simulink model "binary_counter"  (R2022b)
settings: Solver=VariableStepAuto  StartTime=0.0  StopTime=inf  RelTol=1e-3
libraries: simulink_extras x5
settings Model: PacingRate=0.900000  Creator=F1  LastModifiedBy=Namratha
settings SolverCC: AlgebraicLoopSolver=TrustRegion
settings OptimizationCC: BooleanDataType=off
settings DebuggingCC: UnconnectedInputMsg=warning  UnconnectedOutputMsg=warning  UnconnectedLineMsg=warning  SFMachineParentedDataDiag=warning
settings ModelReferenceCC: EnableRefExpFcnMdlSchedulingChecks=on

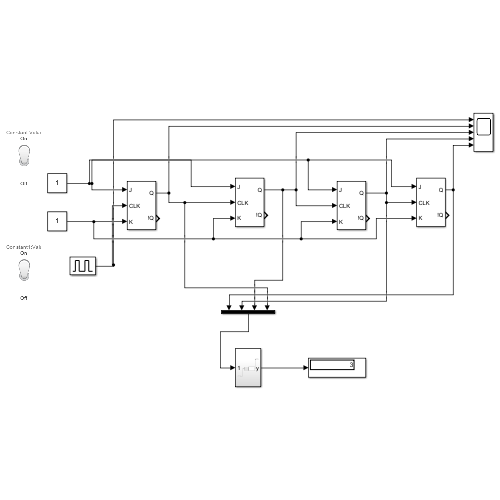
[thumbnail: Simulink's stored preview of the top-level diagram]
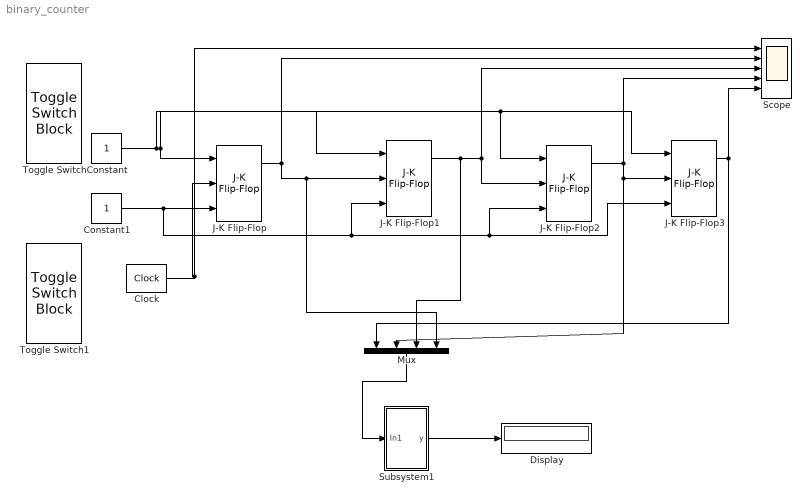
== system binary_counter ==
  Clock : simulink_extras/Flip Flops/Clock  period=2
  Constant : Constant
  Constant1 : Constant
  Display : Display
  J-K Flip-Flop{,1..3} (4 alike) : simulink_extras/Flip Flops/J-K Flip-Flop  initial_condition=0
  Mux : Mux
  Scope : Scope  NumInputPorts=5
  Subsystem1 : Subsystem
  Toggle Switch : ToggleSwitchBlock
      settings: Values={{'Off', 'On'}, [0 1]}
  Toggle Switch1 : ToggleSwitchBlock
      settings: Values={{'Off', 'On'}, [0 1]}
  wires:
  Constant/1 -> J-K Flip-Flop3/1, J-K Flip-Flop2/1, J-K Flip-Flop/1, J-K Flip-Flop1/1
  Constant1/1 -> J-K Flip-Flop3/3, J-K Flip-Flop2/3, J-K Flip-Flop1/3, J-K Flip-Flop/3
  Clock/1 -> J-K Flip-Flop/2, Scope/1
  J-K Flip-Flop/1 -> Scope/2, Mux/4, J-K Flip-Flop1/2
  J-K Flip-Flop1/1 -> J-K Flip-Flop2/2, Scope/3, Mux/3
  J-K Flip-Flop2/1 -> J-K Flip-Flop3/2, Mux/2, Scope/4
  Mux/1 -> Subsystem1/1(In1)
  Subsystem1/1(y) -> Display/1
  J-K Flip-Flop3/1 -> Scope/5, Mux/1

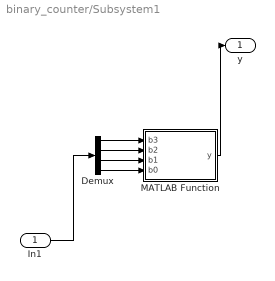
== system binary_counter/Subsystem1 ==
  In1 : Inport
  Demux : Demux
  MATLAB Function : MATLAB Function  TreatAsAtomicUnit=on
  y : Outport
  wires:
  Demux/3 -> MATLAB Function/3(b1)
  Demux/1 -> MATLAB Function/1(b3)
  Demux/2 -> MATLAB Function/2(b2)
  Demux/4 -> MATLAB Function/4(b0)
  MATLAB Function/1(y) -> y/1
  In1/1 -> Demux/1

== matlab function binary_counter/Subsystem1/MATLAB Function ==
  data: b3 input; y output; b2 input; b1 input; b0 input
function y = fcn( b3   , b2   , b1    , b0    )
y =  b3*2^3 + b2*2^2 + b1*2^1 + b0*2^0 ;
end
